simulink model "Driver_CS9"  (Simulink 7.8)
settings: Solver=ode45  SolverMode=SingleTasking  StartTime=0  StopTime=30  FixedStep=0.002  RelTol=1e-3  AbsTol=1e-6
libraries: Solver_SF x1
settings Model: Creator=dhall  LastModifiedBy=bduprey  ExtModeTrigMode=oneshot  ExtModeArmWhenConnect=off
settings DataIOCC: LimitDataPoints=off  SignalLoggingName=sigsOut
settings OptimizationCC: BooleanDataType=off  InitFltsAndDblsToZero=on
settings DebuggingCC: SaveWithParameterizedLinksMsg=none  SignalResolutionControl=TryResolveAllWithWarning  SolverPrmCheckMsg=none  MultiTaskDSMMsg=warning  MultiTaskCondExecSysMsg=none  FcnCallInpInsideContextMsg=Use local settings  StrictBusMsg=None
settings HardwareCC: TargetUnknown=on
settings RTWCC: TemplateMakefile=grt_vc.tmf  IncludeERTFirstTime=on
settings GRTTargetCC: TargetFcnLib=ansi_tfl_tmw.mat  ModelReferenceCompliant=off  MatFileLogging=off

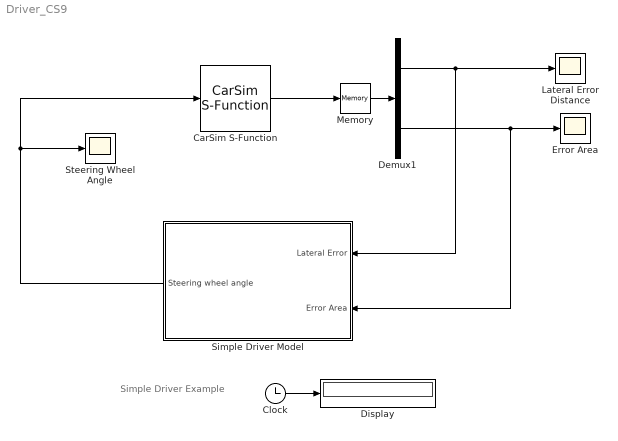
== system Driver_CS9 ==
  note: Simple Driver Example
  CarSim S-Function : Solver_SF/CarSim S-Function  Priority=1  SIMFILE=simfile.sim
  Clock : Clock
  Demux1 : Demux  Outputs=[5 5]
  Display : Display
      settings: Format=bank  Decimation=100
  Error Area : Scope
      settings: TickLabels=on  TimeRange=30  YMin=-6.864406779661017  YMax=6.525423728813561  DataFormat=Array  Decimation=10
  Lateral Error Distance : Scope
      settings: TickLabels=on  TimeRange=30  YMin=-1.196261682242991  YMax=1.308411214953271  DataFormat=Array  Decimation=10
  Memory : Memory
  Simple Driver Model : Subsystem  mask{SENSOR=3, AREA=10, LATERAL=5}
      mask prompts: SENSOR "Selected Sensor"; AREA "Gain of Area Error"; LATERAL "Gain of Lateral Error"
  Steering Wheel Angle : Scope
      settings: TickLabels=on  TimeRange=30  YMin=-50  YMax=50  DataFormat=Array  Decimation=10
  wires:
  CarSim S-Function/1 -> Memory/1
  Demux1/1 -> Simple Driver Model/1(Lateral Error), Lateral Error Distance/1
  Demux1/2 -> Simple Driver Model/2(Error Area), Error Area/1
  Simple Driver Model/1(Steering wheel angle) -> Steering Wheel Angle/1, CarSim S-Function/1
  Clock/1 -> Display/1
  Memory/1 -> Demux1/1

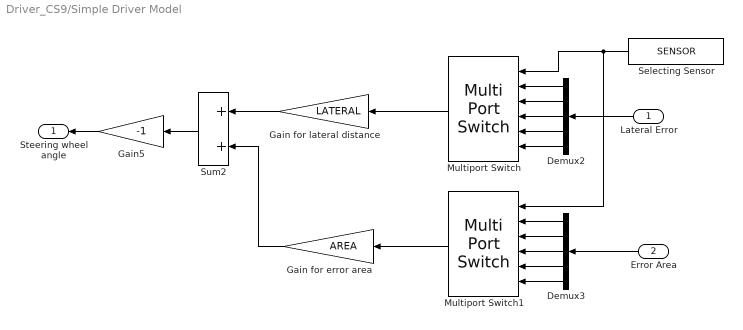
== system Driver_CS9/Simple Driver Model ==
  Lateral Error : Inport
  Error Area : Inport  Port=2
  Demux2 : Demux  Outputs=5
  Demux3 : Demux  Outputs=5
  Gain for error area : Gain  Gain=AREA  SaturateOnIntegerOverflow=on  OutDataTypeStr=Inherit: Same as input  ParamDataTypeStr=Inherit: Same as input
  Gain for lateral distance : Gain  Gain=LATERAL  SaturateOnIntegerOverflow=on  OutDataTypeStr=Inherit: Same as input  ParamDataTypeStr=Inherit: Same as input
  Gain5 : Gain  Gain=-1  SaturateOnIntegerOverflow=on  OutDataTypeStr=Inherit: Same as input  ParamDataTypeStr=Inherit: Same as input
  Multiport Switch : MultiPortSwitch  Inputs=5  zeroidx=off  SaturateOnIntegerOverflow=on  InputSameDT=on
  Multiport Switch1 : MultiPortSwitch  Inputs=5  zeroidx=off  SaturateOnIntegerOverflow=on  InputSameDT=on
  Selecting Sensor : Constant  Value=SENSOR
  Sum2 : Sum  SaturateOnIntegerOverflow=on  InputSameDT=on  OutDataTypeStr=Inherit: Same as first input
  Steering wheel angle : Outport  InitialOutput=0
  wires:
  Demux2/1 -> Multiport Switch/2
  Demux2/2 -> Multiport Switch/3
  Demux2/3 -> Multiport Switch/4
  Demux2/4 -> Multiport Switch/5
  Demux2/5 -> Multiport Switch/6
  Demux3/1 -> Multiport Switch1/2
  Demux3/2 -> Multiport Switch1/3
  Demux3/3 -> Multiport Switch1/4
  Demux3/5 -> Multiport Switch1/6
  Demux3/4 -> Multiport Switch1/5
  Lateral Error/1 -> Demux2/1
  Error Area/1 -> Demux3/1
  Selecting Sensor/1 -> Multiport Switch/1, Multiport Switch1/1
  Multiport Switch/1 -> Gain for lateral distance/1
  Multiport Switch1/1 -> Gain for error area/1
  Gain for lateral distance/1 -> Sum2/1
  Gain for error area/1 -> Sum2/2
  Sum2/1 -> Gain5/1
  Gain5/1 -> Steering wheel angle/1
